simulink model "BPSKmodem"  (R2013a)
settings: Solver=ode45  StartTime=0.0  StopTime=100/1200  RelTol=1e-3
undefined symbols (not defined in the file): DiscIntNeverNeededParam
libraries: simulink_extras x8, dsparch4 x5, simulink x2, commnoisgen2 x1, commchan3 x1, commrandsrc2 x1, commsynccomp2 x1, commsink2 x1
settings Model: Creator=Cedric  LastModifiedBy=Cedric

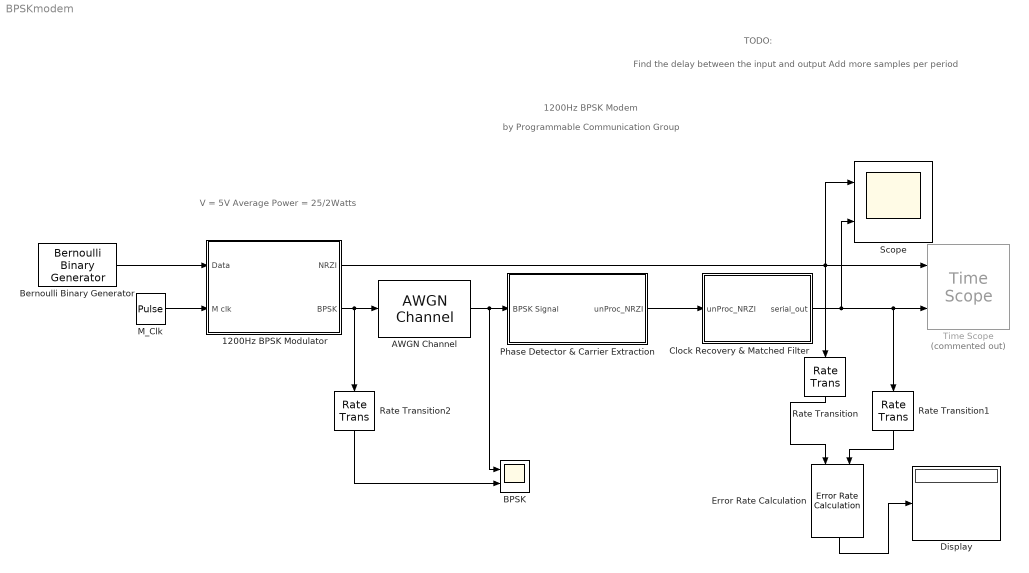
== system BPSKmodem ==
  note: V = 5V
      | Average Power = 25/2Watts
  note: Find the delay between the input and output
      | Add more samples per period
  note: TODO:
  note: 1200Hz BPSK Modem
  note: by Programmable Communication Group
  1200Hz BPSK Modulator : Subsystem
  AWGN Channel : commchan3/AWGN Channel  InputProcessing=Columns as channels (frame based)  seed=randseed  noiseMode=Variance from mask  EbNodB=10  EsNodB=10  SNRdB=-1  bitsPerSym=1  Ps=25/2  Tsym=1  variance=1
  BPSK : Scope  NumInputPorts=2
      settings: ShowLegends=on  YMin=-5~-5  YMax=5~5  SaveName=ScopeData2
  Bernoulli Binary Generator : commrandsrc2/Bernoulli Binary Generator  P=0.5  seed=randseed  Ts=1/600  frameBased=off  sampPerFrame=1  orient=on  outDataType=boolean
  Clock Recovery & Matched Filter : Subsystem
  Display : Display
  Error Rate Calculation : commsink2/Error Rate Calculation  N=1  st_delay=0  cp_mode=Entire frame  subframe=[]  PMode=Port  WsName=ErrorVec  RsMode2=off  stop=off  numErr=100  maxBits=1e6
  M_Clk : DiscretePulseGenerator  Period=4  PulseWidth=2  SampleTime=1/(19200*4)
  Phase Detector & Carrier Extraction : Subsystem
  Rate Transition : RateTransition  OutPortSampleTime=1/(1200)
  Rate Transition1 : RateTransition  OutPortSampleTime=1/(1200)
  Rate Transition2 : RateTransition  OutPortSampleTime=1/(256*1200)
  Scope : Scope  NumInputPorts=2
      settings: ShowLegends=on  YMin=-5~-5  YMax=5~5
  Time Scope : TimeScope  Commented=on  NumInputPorts=2  DefaultConfigurationName=spbscopes.TimeScopeBlockCfg
      settings: CopyFcn=scopeextensions.ScopeBlock.callback(gcbh, 'onBlockCopy', gcbh);  DeleteFcn=scopeextensions.ScopeBlock.callback(gcbh, 'onBlockDelete');  PreSaveFcn=scopeextensions.ScopeBlock.callback(gcbh, 'onModelSave');  NameChangeFcn=scopeextensions.ScopeBlock.callback(gcbh, 'onBlockRename');  CloseFcn=scopeextensions.ScopeBlock.callback(gcbh, 'onBlockClose');  PreDeleteFcn=scopeextensions.ScopeBlock.callback(gcbh, 'onBlockPreDelete');
  wires:
  Bernoulli Binary Generator/1 -> 1200Hz BPSK Modulator/1(Data)
  M_Clk/1 -> 1200Hz BPSK Modulator/2(M clk)
  Phase Detector & Carrier Extraction/1(unProc_NRZI) -> Clock Recovery & Matched Filter/1(unProc_NRZI)
  Clock Recovery & Matched Filter/1(serial_out) -> Time Scope/2, Rate Transition1/1, Scope/2
  1200Hz BPSK Modulator/1(NRZI) -> Scope/1, Time Scope/1, Rate Transition/1
  Error Rate Calculation/1 -> Display/1
  Rate Transition/1 -> Error Rate Calculation/1
  Rate Transition1/1 -> Error Rate Calculation/2
  1200Hz BPSK Modulator/2(BPSK) -> AWGN Channel/1, Rate Transition2/1
  Rate Transition2/1 -> BPSK/2
  AWGN Channel/1 -> BPSK/1, Phase Detector & Carrier Extraction/1(BPSK Signal)

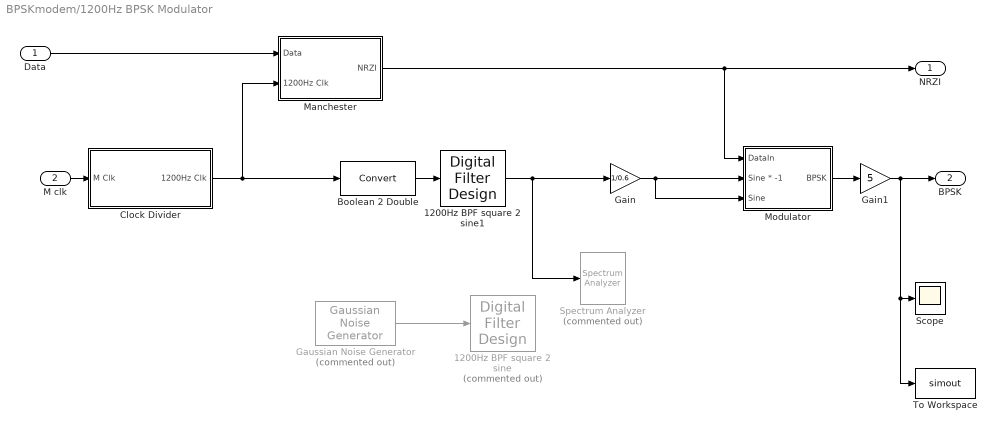
== system BPSKmodem/1200Hz BPSK Modulator ==
  Data : Inport
  M clk : Inport  Port=2
  1200Hz BPF square 2 sine : dsparch4/Digital Filter Design  Commented=on  mwdsp_browser_bugfix_var=off
  1200Hz BPF square 2 sine1 : dsparch4/Digital Filter Design  mwdsp_browser_bugfix_var=off
  Boolean 2 Double : DataTypeConversion  SampleTime=1/(19200*4)
  Clock Divider : Subsystem
  Gain : Gain  Gain=1/0.6
  Gain1 : Gain  Gain=5
  Gaussian Noise Generator : commnoisgen2/Gaussian Noise Generator  Commented=on  m=0  d=1  s=randseed  Ts=1/76800  frameBased=off  sampPerFrame=1  orient=off  outDataType=double
  Manchester : Subsystem
  Modulator : Subsystem
  Scope : Scope
      settings: YMin=-3e-08  YMax=3e-08
  Spectrum Analyzer : SpectrumAnalyzer  Commented=on
      settings: CopyFcn=scopeextensions.ScopeBlock.callback(gcbh, 'onBlockCopy', gcbh);  DeleteFcn=scopeextensions.ScopeBlock.callback(gcbh, 'onBlockDelete');  PreSaveFcn=scopeextensions.ScopeBlock.callback(gcbh, 'onModelSave');  NameChangeFcn=scopeextensions.ScopeBlock.callback(gcbh, 'onBlockRename');  CloseFcn=scopeextensions.ScopeBlock.callback(gcbh, 'onBlockClose');  PreDeleteFcn=scopeextensions.ScopeBlock.callback(gcbh, 'onBlockPreDelete');
  To Workspace : ToWorkspace  VariableName=simout  SampleTime=-1  SaveFormat=Timeseries
  NRZI : Outport
  BPSK : Outport  Port=2
  wires:
  Modulator/1(BPSK) -> Gain1/1
  Gain/1 -> Modulator/3(Sine), Modulator/2(Sine * -1)
  Clock Divider/1(1200Hz Clk) -> Manchester/2(1200Hz Clk), Boolean 2 Double/1
  M clk/1 -> Clock Divider/1(M Clk)
  Data/1 -> Manchester/1(Data)
  Manchester/1(NRZI) -> NRZI/1, Modulator/1(DataIn)
  Gaussian Noise Generator/1 -> 1200Hz BPF square 2 sine/1
  Boolean 2 Double/1 -> 1200Hz BPF square 2 sine1/1
  1200Hz BPF square 2 sine1/1 -> Spectrum Analyzer/1, Gain/1
  Gain1/1 -> To Workspace/1, Scope/1, BPSK/1

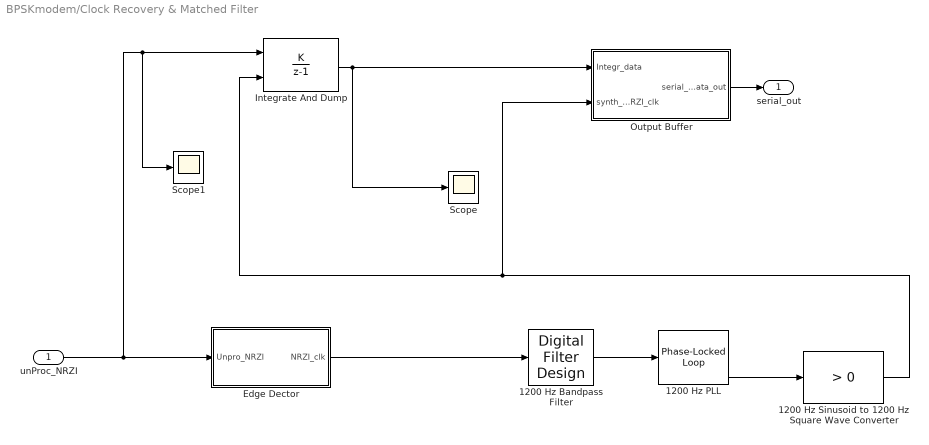
== system BPSKmodem/Clock Recovery & Matched Filter ==
  unProc_NRZI : Inport
  "1200 Hz Bandpass Filter " : dsparch4/Digital Filter Design  mwdsp_browser_bugfix_var=off
  1200 Hz PLL : commsynccomp2/Phase-Locked Loop  Fn="[3.0002  0  40002]"  Fd="[1   67.46   2270.9   40002]"  Kvco=1  Fc=1200  Ph=3.14  Ac=1
  1200 Hz Sinusoid to 1200 Hz Square Wave Converter : simulink/Logic and Bit Operations/Compare To Zero  relop=>  OutDataTypeStr=boolean
  Edge Dector : Subsystem
  Integrate And Dump : DiscreteIntegrator  IntegratorMethod=Accumulation: Forward Euler  ExternalReset=rising  InitialCondition=1  SampleTime=1/(1200*64)  ICPrevOutput=DiscIntNeverNeededParam  ICPrevScaledInput=DiscIntNeverNeededParam
  Output Buffer : Subsystem
  Scope : Scope
      settings: SaveName=ScopeData4
  Scope1 : Scope
      settings: YMin=-0.5  YMax=1.5  SaveName=ScopeData5
  serial_out : Outport
  wires:
  Output Buffer/1(serial_data_out) -> serial_out/1
  unProc_NRZI/1 -> Edge Dector/1(Unpro_NRZI), Scope1/1, Integrate And Dump/1
  1200 Hz Sinusoid to 1200 Hz Square Wave Converter/1 -> Output Buffer/2(synth_NRZI_clk), Integrate And Dump/2
  1200 Hz PLL/3 -> 1200 Hz Sinusoid to 1200 Hz Square Wave Converter/1
  "1200 Hz Bandpass Filter "/1 -> 1200 Hz PLL/1
  Edge Dector/1(NRZI_clk) -> "1200 Hz Bandpass Filter "/1
  Integrate And Dump/1 -> Scope/1, Output Buffer/1(Integr_data)

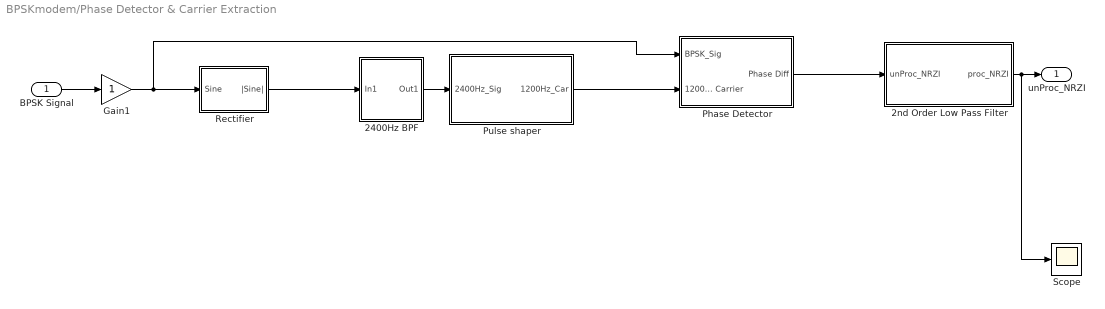
== system BPSKmodem/Phase Detector & Carrier Extraction ==
  BPSK Signal : Inport
  2400Hz BPF : Subsystem
  2nd Order Low Pass Filter : Subsystem
  Gain1 : Gain
  Phase Detector : Subsystem
  Pulse shaper : Subsystem
  Rectifier : Subsystem
  Scope : Scope
      settings: YMin=-0.5  YMax=1.5  SaveName=ScopeData3
  unProc_NRZI : Outport
  wires:
  BPSK Signal/1 -> Gain1/1
  Gain1/1 -> Phase Detector/1(BPSK_Sig), Rectifier/1(Sine)
  2nd Order Low Pass Filter/1(proc_NRZI) -> Scope/1, unProc_NRZI/1
  Rectifier/1(|Sine|) -> 2400Hz BPF/1(In1)
  2400Hz BPF/1(Out1) -> Pulse shaper/1(2400Hz_Sig)
  Phase Detector/1(Phase Diff) -> 2nd Order Low Pass Filter/1(unProc_NRZI)
  Pulse shaper/1(1200Hz_Car) -> Phase Detector/2(1200Hz Carrier)

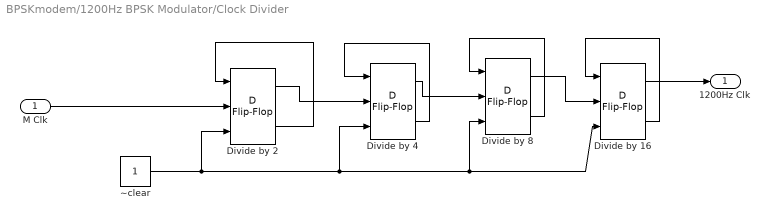
== system BPSKmodem/1200Hz BPSK Modulator/Clock Divider ==
  M Clk : Inport
  Divide by {2,4,8,16} (4 alike) : simulink_extras/Flip Flops/D Flip-Flop
  ~clear : Constant
  1200Hz Clk : Outport
  wires:
  M Clk/1 -> Divide by 2/2
  ~clear/1 -> Divide by 16/3, Divide by 8/3, Divide by 4/3, Divide by 2/3
  Divide by 2/2 -> Divide by 2/1
  Divide by 2/1 -> Divide by 4/2
  Divide by 4/2 -> Divide by 4/1
  Divide by 4/1 -> Divide by 8/2
  Divide by 8/2 -> Divide by 8/1
  Divide by 8/1 -> Divide by 16/2
  Divide by 16/1 -> 1200Hz Clk/1
  Divide by 16/2 -> Divide by 16/1

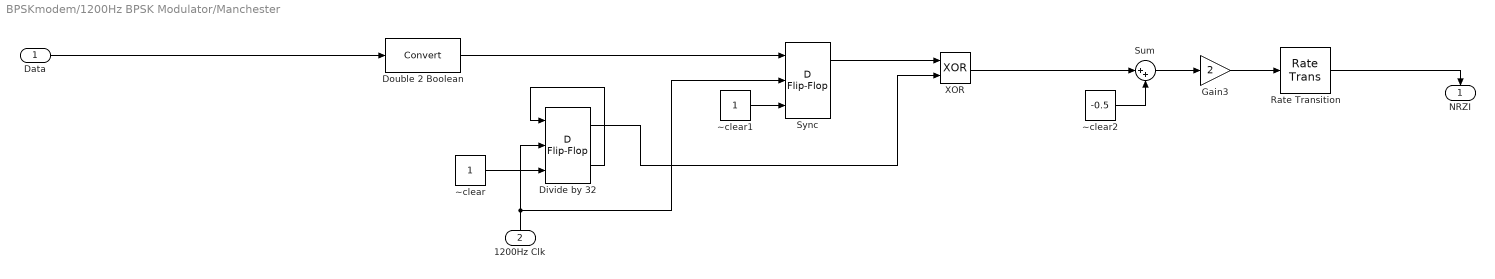
== system BPSKmodem/1200Hz BPSK Modulator/Manchester ==
  Data : Inport
  1200Hz Clk : Inport  Port=2
  Divide by 32 : simulink_extras/Flip Flops/D Flip-Flop
  Double 2 Boolean : DataTypeConversion  SampleTime=1/(19200*4)
  Gain3 : Gain  Gain=2
  Rate Transition : RateTransition
  Sum : Sum  Inputs=|++
  Sync : simulink_extras/Flip Flops/D Flip-Flop
  XOR : Logic  Operator=XOR  AllPortsSameDT=off  OutDataTypeStr=boolean
  ~clear : Constant
  ~clear1 : Constant
  ~clear2 : Constant  Value=-0.5
  NRZI : Outport
  wires:
  Sync/1 -> XOR/1
  XOR/1 -> Sum/1
  Gain3/1 -> Rate Transition/1
  Divide by 32/2 -> Divide by 32/1
  Divide by 32/1 -> XOR/2
  Rate Transition/1 -> NRZI/1
  Data/1 -> Double 2 Boolean/1
  ~clear1/1 -> Sync/3
  Double 2 Boolean/1 -> Sync/1
  Sum/1 -> Gain3/1
  ~clear2/1 -> Sum/2
  ~clear/1 -> Divide by 32/3
  1200Hz Clk/1 -> Divide by 32/2, Sync/2

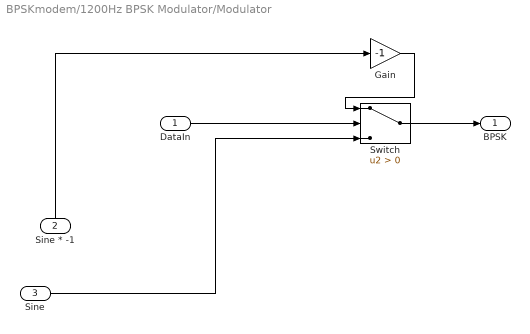
== system BPSKmodem/1200Hz BPSK Modulator/Modulator ==
  DataIn : Inport
  Sine * -1 : Inport  Port=2
  Sine : Inport  Port=3
  Gain : Gain  Gain=-1
  Switch : Switch  Criteria=u2 > Threshold
  BPSK : Outport
  wires:
  DataIn/1 -> Switch/2
  Sine/1 -> Switch/3
  Sine * -1/1 -> Gain/1
  Gain/1 -> Switch/1
  Switch/1 -> BPSK/1

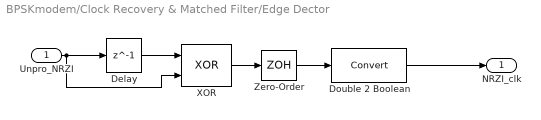
== system BPSKmodem/Clock Recovery & Matched Filter/Edge Dector ==
  Unpro_NRZI : Inport
  Delay : Delay  DelayLength=1  SampleTime=1/(1200*64)
  Double 2 Boolean : DataTypeConversion
  XOR : Logic  Operator=XOR  IconShape=distinctive  AllPortsSameDT=off  OutDataTypeStr=boolean  SampleTime=1/(1200*64)
  Zero-Order : ZeroOrderHold  SampleTime=-1
  NRZI_clk : Outport
  wires:
  Zero-Order/1 -> Double 2 Boolean/1
  Double 2 Boolean/1 -> NRZI_clk/1
  XOR/1 -> Zero-Order/1
  Delay/1 -> XOR/1
  Unpro_NRZI/1 -> XOR/2, Delay/1

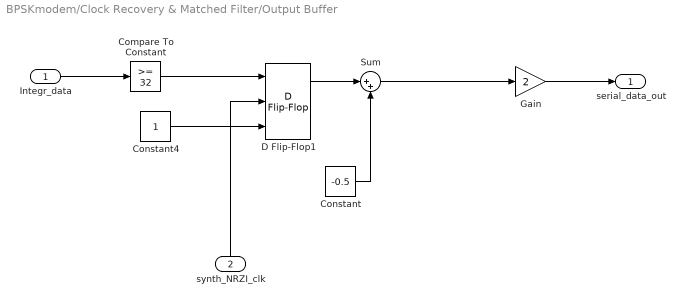
== system BPSKmodem/Clock Recovery & Matched Filter/Output Buffer ==
  Integr_data : Inport
  synth_NRZI_clk : Inport  Port=2
  Compare To Constant : simulink/Logic and Bit Operations/Compare To Constant  relop=>=  const=32  OutDataTypeStr=boolean
  Constant : Constant  Value=-0.5
  Constant4 : Constant
  D Flip-Flop1 : simulink_extras/Flip Flops/D Flip-Flop
  Gain : Gain  Gain=2
  Sum : Sum  Inputs=|++
  serial_data_out : Outport
  wires:
  Compare To Constant/1 -> D Flip-Flop1/1
  Integr_data/1 -> Compare To Constant/1
  Constant4/1 -> D Flip-Flop1/3
  synth_NRZI_clk/1 -> D Flip-Flop1/2
  Gain/1 -> serial_data_out/1
  D Flip-Flop1/1 -> Sum/1
  Sum/1 -> Gain/1
  Constant/1 -> Sum/2

== system BPSKmodem/Phase Detector & Carrier Extraction/2400Hz BPF ==
  In1 : Inport
  BPF 2400Hz Noise : dsparch4/Digital Filter Design  mwdsp_browser_bugfix_var=off
  Out1 : Outport
  wires:
  In1/1 -> BPF 2400Hz Noise/1
  BPF 2400Hz Noise/1 -> Out1/1

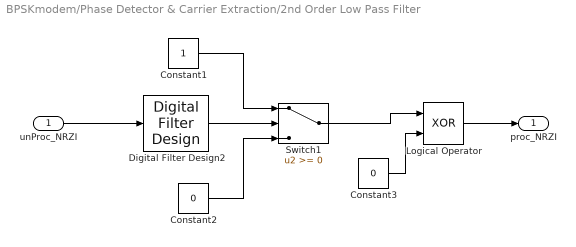
== system BPSKmodem/Phase Detector & Carrier Extraction/2nd Order Low Pass Filter ==
  unProc_NRZI : Inport
  Constant1 : Constant
  Constant2 : Constant  Value=0
  Constant3 : Constant  Value=0
  Digital Filter Design2 : dsparch4/Digital Filter Design  mwdsp_browser_bugfix_var=off
  Logical Operator : Logic  Operator=XOR  AllPortsSameDT=off  OutDataTypeStr=boolean
  Switch1 : Switch
  proc_NRZI : Outport
  wires:
  Logical Operator/1 -> proc_NRZI/1
  Digital Filter Design2/1 -> Switch1/2
  Constant1/1 -> Switch1/1
  Constant2/1 -> Switch1/3
  Switch1/1 -> Logical Operator/1
  Constant3/1 -> Logical Operator/2
  unProc_NRZI/1 -> Digital Filter Design2/1

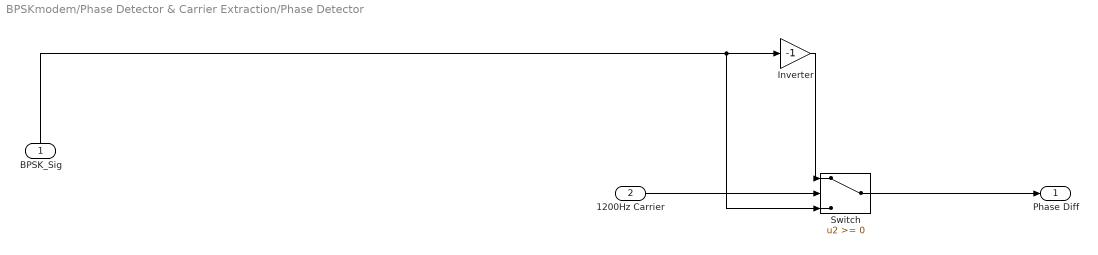
== system BPSKmodem/Phase Detector & Carrier Extraction/Phase Detector ==
  BPSK_Sig : Inport
  1200Hz Carrier : Inport  Port=2
  Inverter : Gain  Gain=-1
  Switch : Switch
  Phase Diff : Outport
  wires:
  Inverter/1 -> Switch/1
  Switch/1 -> Phase Diff/1
  1200Hz Carrier/1 -> Switch/2
  BPSK_Sig/1 -> Switch/3, Inverter/1

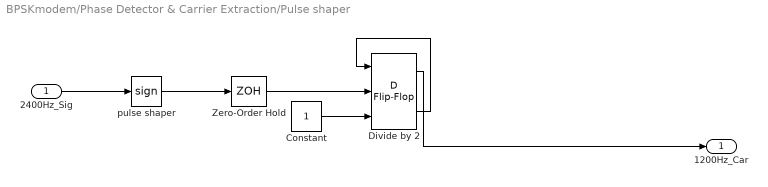
== system BPSKmodem/Phase Detector & Carrier Extraction/Pulse shaper ==
  2400Hz_Sig : Inport
  Constant : Constant
  Divide by 2 : simulink_extras/Flip Flops/D Flip-Flop
  Zero-Order Hold : ZeroOrderHold  SampleTime=-1
  pulse shaper : Signum
  1200Hz_Car : Outport
  wires:
  pulse shaper/1 -> Zero-Order Hold/1
  Zero-Order Hold/1 -> Divide by 2/2
  Divide by 2/2 -> Divide by 2/1
  Constant/1 -> Divide by 2/3
  Divide by 2/1 -> 1200Hz_Car/1
  2400Hz_Sig/1 -> pulse shaper/1

== system BPSKmodem/Phase Detector & Carrier Extraction/Rectifier ==
  Sine : Inport
  Product : Product
  |Sine| : Outport
  wires:
  Sine/1 -> Product/1, Product/2
  Product/1 -> |Sine|/1
